simulink model "Watermark"  (R2021a)
settings: Solver=VariableStepAuto  StartTime=0.0  StopTime=tsim  RelTol=1e-3
values from neighbouring files (symbols this model uses):
  attack_DoS = 1    [main.m]
  attack_sat = 0    [main.m]
  delay = 700    [main.m]
  gamma1 = 0.70    (= 0.7)    [main.m]
  gamma2 = 0.60    (= 0.6)    [main.m]
  r1 = kc*h01    [main.m]
  r2 = kc*h02    [main.m]
  seuil_H0 = chi2inv(1-PFA, n_chi2 * timeWindow)    [main.m]
  SigmaInv = inv(Sigma)    [main.m]
  ta = 0.6*tsim    (= 1200)    [main.m]
undefined symbols (not defined in the file or in its folder): A1, a1, A2, a2, A3, a3, A4, a4, Adlin, Bdlin, C, Cdlin, g, K, k1, k2, L, m, n, sat_hmax, sat_hmin, sat_vmax, sat_vmin, sigma2_b, Ts, v01, v02, xd0
libraries: simulink x3, dspsrcs4 x2, commfilt2 x1
settings Model: Creator=aperodou  LastModifiedBy=Arthur
settings SolverCC: AlgebraicLoopSolver=TrustRegion
settings DebuggingCC: SFMachineParentedDataDiag=warning

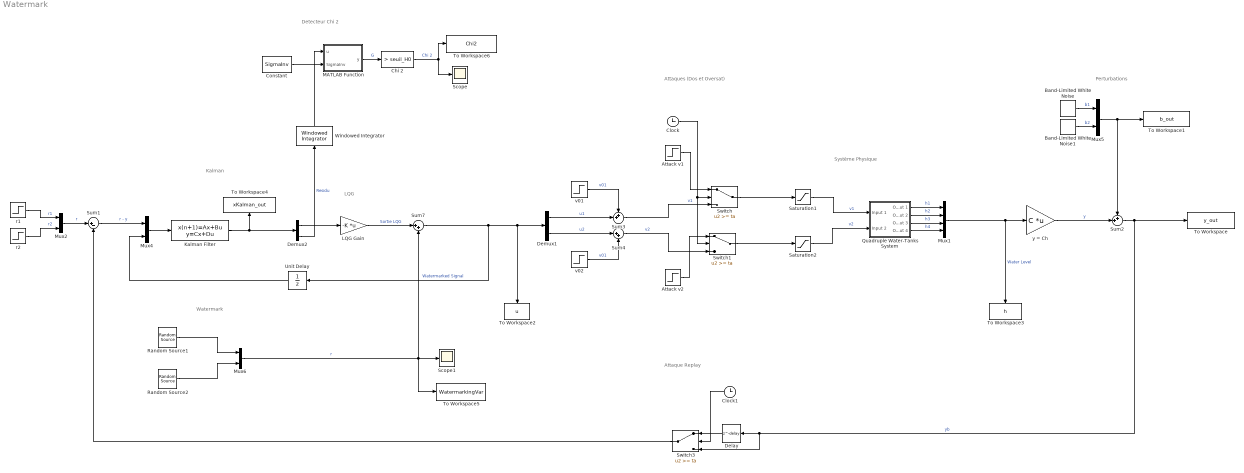
== system Watermark ==
  note: Attaques
      | (Dos et Oversat)
  note: Kalman
  note: Perturbations
  note: Système Physique
  note: Detecteur Chi 2
  note: LQG
  note: Attaque Replay
  note: Watermark
  Attack v1 : Step  Time=0  After=attack_DoS*0 + attack_sat*sat_vmax  SampleTime=0
  Attack v2 : Step  Time=0  After=attack_DoS*0 + attack_sat*sat_vmax  SampleTime=0
  Band-Limited White Noise : simulink/Sources/Band-Limited White Noise  Cov=[ sigma2_b ]  Ts=Ts  seed=[23341]
  Band-Limited White Noise1 : simulink/Sources/Band-Limited White Noise  Cov=[ sigma2_b]  Ts=Ts  seed=[20000]
  Chi 2 : simulink/Logic and Bit Operations/Compare To Constant  relop=>  const=seuil_H0  OutDataTypeStr=boolean
  Clock : Clock
  Clock1 : Clock
  Constant : Constant  Value=SigmaInv
  Delay : Delay  DelayLength=delay  InitialCondition=0
  Demux1 : Demux  Outputs=2
  Demux2 : Demux  Outputs=2
  Kalman Filter : DiscreteStateSpace  A=Adlin  B=[zeros(n,m) -Bdlin]  C=[eye(n) - L*Cdlin ; -Cdlin]  D=[L zeros(n,m) ; eye(m) zeros(m,m)]  InitialCondition=xd0  SampleTime=Ts
  LQG Gain : Gain  Gain=-K  Multiplication=Matrix(K*u) (u vector)
  MATLAB Function : MATLAB Function  TreatAsAtomicUnit=on
  Mux1 : Mux
  Mux{2,4..6} (4 alike) : Mux  Inputs=2
  Quadruple Water-Tanks System : Subsystem
  Random Source1 : dspsrcs4/Random Source  SrcType=Gaussian  NormMethod=Ziggurat  CltLength=12  MinVal=0  MaxVal=1  MeanVal=0  VarVal=varW  RepMode=Not repeatable  rawSeed=1  IsInherit=off  SampMode=Discrete  SampTime=1  SampFrame=1  DataType=Double  OutComplex=Real  OutputFrames=off
  Random Source2 : dspsrcs4/Random Source  SrcType=Gaussian  NormMethod=Ziggurat  CltLength=12  MinVal=0  MaxVal=1  MeanVal=0  VarVal=varW  RepMode=Not repeatable  rawSeed=1  IsInherit=off  SampMode=Discrete  SampTime=1  SampFrame=1  DataType=Double  OutComplex=Real  OutputFrames=off
  Saturation1 : Saturate  UpperLimit=sat_vmax  LowerLimit=sat_vmin
  Saturation2 : Saturate  UpperLimit=sat_vmax  LowerLimit=sat_vmin
  Scope : Scope
  Scope1 : Scope
  Sum1 : Sum  Inputs=|+-  SaturateOnIntegerOverflow=on
  Sum2 : Sum  Inputs=++|  SaturateOnIntegerOverflow=on
  Sum3 : Sum  Inputs=++|  SaturateOnIntegerOverflow=on
  Sum4 : Sum  Inputs=|++  SaturateOnIntegerOverflow=on
  Sum7 : Sum  Inputs=|++  SaturateOnIntegerOverflow=on
  Switch : Switch  Threshold=ta
  Switch1 : Switch  Threshold=ta
  Switch3 : Switch  Threshold=ta
  To Workspace : ToWorkspace  VariableName=y_out  SaveFormat=Timeseries  SampleTime=-1
  To Workspace1 : ToWorkspace  VariableName=b_out  SaveFormat=Timeseries  SampleTime=-1
  To Workspace2 : ToWorkspace  VariableName=u  SampleTime=-1
  To Workspace3 : ToWorkspace  VariableName=h  SampleTime=-1
  To Workspace4 : ToWorkspace  VariableName=xKalman_out  SaveFormat=Timeseries  SampleTime=-1
  To Workspace5 : ToWorkspace  VariableName=WatermarkingVar  SaveFormat=Timeseries  SampleTime=-1
  To Workspace6 : ToWorkspace  VariableName=Chi2  SampleTime=-1
  Unit Delay : UnitDelay  SampleTime=Ts  HasFrameUpgradeWarning=on
  Windowed Integrator : commfilt2/Windowed Integrator  integperiod=timeWindow  roundingMode=Floor  overflowMode=off  coeffDataTypeStr=Inherit: Same word length as input  coeffMin=[]  coeffMax=[]  coeffLastDataTypeStr=Inherit: Same word length as input  accumDataTypeStr=Inherit: Same as product output  accumLastDataTypeStr=Inherit: Same as product output  outputDataTypeStr=Inherit: Same as accumulator  outputMin=[]  outputMax=[]  outputLastDataTypeStr=Inherit: Same as accumulator
      settings: SourceProductBaseCode=CM
  r1 : Step  Time=0  After=r1  SampleTime=0
  r2 : Step  Time=0  After=r2  SampleTime=0
  v01 : Step  Time=0  After=v01  SampleTime=Ts
  v02 : Step  Time=0  After=v02  SampleTime=Ts
  y = Ch : Gain  Gain=C  Multiplication=Matrix(K*u) (u vector)
  wires:
  Quadruple Water-Tanks System/1(Output 1) -> Mux1/1  "h1"
  Quadruple Water-Tanks System/2(Output 2) -> Mux1/2  "h2"
  Quadruple Water-Tanks System/3(Output 3) -> Mux1/3  "h3"
  Quadruple Water-Tanks System/4(Output 4) -> Mux1/4  "h4"
  Mux1/1 -> y = Ch/1, To Workspace3/1  "Water Level"
  Mux2/1 -> Sum1/1  "r"
  Clock/1 -> Switch1/2, Switch/2
  Sum2/1 -> To Workspace/1, Switch3/3, Delay/1  "yb"
  y = Ch/1 -> Sum2/2  "y"
  r2/1 -> Mux2/2  "r2"
  r1/1 -> Mux2/1  "r1"
  Kalman Filter/1 -> Demux2/1, To Workspace4/1
  LQG Gain/1 -> Sum7/1  "Sortie LQG"
  Mux4/1 -> Kalman Filter/1
  Sum1/1 -> Mux4/1  "r - y"
  Unit Delay/1 -> Mux4/2
  Saturation1/1 -> Quadruple Water-Tanks System/1(Input 1)  "v1"
  Saturation2/1 -> Quadruple Water-Tanks System/2(Input 2)  "v2"
  v01/1 -> Sum3/1  "v01"
  Demux1/1 -> Sum3/2  "u1"
  Sum3/1 -> Switch/3  "v1"
  v02/1 -> Sum4/2  "v01"
  Demux1/2 -> Sum4/1  "u2"
  Sum4/1 -> Switch1/3  "v2"
  Band-Limited White Noise/1 -> Mux5/1  "b1"
  Band-Limited White Noise1/1 -> Mux5/2  "b2"
  Mux5/1 -> Sum2/1, To Workspace1/1
  Demux2/1 -> LQG Gain/1
  Constant/1 -> MATLAB Function/2(SigmaInv)
  MATLAB Function/1(y) -> Chi 2/1  "G"
  Demux2/2 -> Windowed Integrator/1  "Residu"
  Chi 2/1 -> To Workspace6/1, Scope/1  "Chi 2"
  Delay/1 -> Switch3/1
  Clock1/1 -> Switch3/2
  Attack v1/1 -> Switch/1
  Attack v2/1 -> Switch1/1
  Switch/1 -> Saturation1/1
  Switch1/1 -> Saturation2/1
  Switch3/1 -> Sum1/2
  Random Source1/1 -> Mux6/1
  Mux6/1 -> To Workspace5/1, Sum7/2, Scope1/1  "r"
  Random Source2/1 -> Mux6/2
  Sum7/1 -> Demux1/1, To Workspace2/1, Unit Delay/1  "Watermarked Signal"
  Windowed Integrator/1 -> MATLAB Function/1(u)

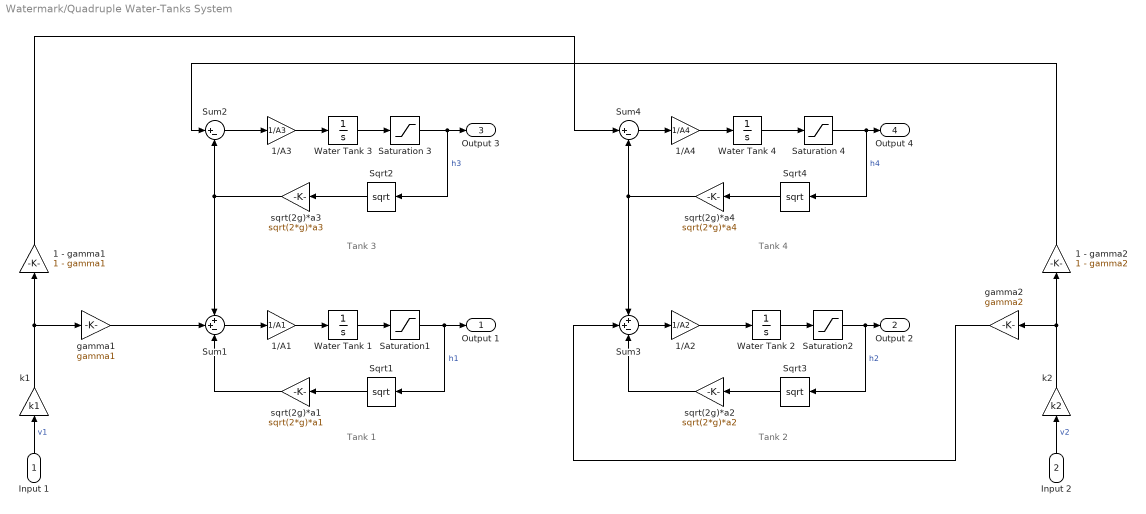
== system Watermark/Quadruple Water-Tanks System ==
  note: Tank 1
  note: Tank 3
  note: Tank 4
  note: Tank 2
  Input 1 : Inport
  Input 2 : Inport  Port=2
  1 - gamma1 : Gain  Gain=1 - gamma1  SaturateOnIntegerOverflow=on  OutDataTypeStr=Inherit: Same as input  ParamDataTypeStr=Inherit: Same as input
  1 - gamma2 : Gain  Gain=1 - gamma2  SaturateOnIntegerOverflow=on  OutDataTypeStr=Inherit: Same as input  ParamDataTypeStr=Inherit: Same as input
  1/A1 : Gain  Gain=1/A1  SaturateOnIntegerOverflow=on  OutDataTypeStr=Inherit: Same as input  ParamDataTypeStr=Inherit: Same as input
  1/A2 : Gain  Gain=1/A2  SaturateOnIntegerOverflow=on  OutDataTypeStr=Inherit: Same as input  ParamDataTypeStr=Inherit: Same as input
  1/A3 : Gain  Gain=1/A3  SaturateOnIntegerOverflow=on  OutDataTypeStr=Inherit: Same as input  ParamDataTypeStr=Inherit: Same as input
  1/A4 : Gain  Gain=1/A4  SaturateOnIntegerOverflow=on  OutDataTypeStr=Inherit: Same as input  ParamDataTypeStr=Inherit: Same as input
  Saturation 3 : Saturate  UpperLimit=sat_hmax  LowerLimit=sat_hmin
  Saturation 4 : Saturate  UpperLimit=sat_hmax  LowerLimit=sat_hmin
  Saturation1 : Saturate  UpperLimit=sat_hmax  LowerLimit=sat_hmin
  Saturation2 : Saturate  UpperLimit=sat_hmax  LowerLimit=sat_hmin
  Sqrt{1..4} (4 alike) : Sqrt  SaturateOnIntegerOverflow=on
  Sum1 : Sum  Inputs=++-  SaturateOnIntegerOverflow=on
  Sum2 : Sum  Inputs=|+-  SaturateOnIntegerOverflow=on
  Sum3 : Sum  Inputs=++-  SaturateOnIntegerOverflow=on
  Sum4 : Sum  Inputs=|+-  SaturateOnIntegerOverflow=on
  Water Tank {1..4} (4 alike) : Integrator
  gamma1 : Gain  Gain=gamma1  SaturateOnIntegerOverflow=on  OutDataTypeStr=Inherit: Same as input  ParamDataTypeStr=Inherit: Same as input
  gamma2 : Gain  Gain=gamma2  SaturateOnIntegerOverflow=on  OutDataTypeStr=Inherit: Same as input  ParamDataTypeStr=Inherit: Same as input
  k1 : Gain  Gain=k1  SaturateOnIntegerOverflow=on  OutDataTypeStr=Inherit: Same as input  ParamDataTypeStr=Inherit: Same as input
  k2 : Gain  Gain=k2  SaturateOnIntegerOverflow=on  OutDataTypeStr=Inherit: Same as input  ParamDataTypeStr=Inherit: Same as input
  sqrt(2g)*a1 : Gain  Gain=sqrt(2*g)*a1  SaturateOnIntegerOverflow=on  OutDataTypeStr=Inherit: Same as input  ParamDataTypeStr=Inherit: Same as input
  sqrt(2g)*a2 : Gain  Gain=sqrt(2*g)*a2  SaturateOnIntegerOverflow=on  OutDataTypeStr=Inherit: Same as input  ParamDataTypeStr=Inherit: Same as input
  sqrt(2g)*a3 : Gain  Gain=sqrt(2*g)*a3  SaturateOnIntegerOverflow=on  OutDataTypeStr=Inherit: Same as input  ParamDataTypeStr=Inherit: Same as input
  sqrt(2g)*a4 : Gain  Gain=sqrt(2*g)*a4  SaturateOnIntegerOverflow=on  OutDataTypeStr=Inherit: Same as input  ParamDataTypeStr=Inherit: Same as input
  Output 1 : Outport  VectorParamsAs1DForOutWhenUnconnected=off
  Output 2 : Outport  Port=2  VectorParamsAs1DForOutWhenUnconnected=off
  Output 3 : Outport  Port=3  VectorParamsAs1DForOutWhenUnconnected=off
  Output 4 : Outport  Port=4  VectorParamsAs1DForOutWhenUnconnected=off
  wires:
  Saturation2/1 -> Sqrt3/1, Output 2/1  "h2"
  Water Tank 2/1 -> Saturation2/1
  Water Tank 4/1 -> Saturation 4/1
  1/A1/1 -> Water Tank 1/1
  Sqrt2/1 -> sqrt(2g)*a3/1
  Saturation1/1 -> Sqrt1/1, Output 1/1  "h1"
  Water Tank 3/1 -> Saturation 3/1
  sqrt(2g)*a3/1 -> Sum2/2, Sum1/1
  sqrt(2g)*a4/1 -> Sum4/2, Sum3/1
  Saturation 3/1 -> Sqrt2/1, Output 3/1  "h3"
  Saturation 4/1 -> Sqrt4/1, Output 4/1  "h4"
  1/A4/1 -> Water Tank 4/1
  Water Tank 1/1 -> Saturation1/1
  Sum1/1 -> 1/A1/1
  Sqrt3/1 -> sqrt(2g)*a2/1
  k1/1 -> 1 - gamma1/1, gamma1/1
  Sqrt4/1 -> sqrt(2g)*a4/1
  k2/1 -> 1 - gamma2/1, gamma2/1
  Sum4/1 -> 1/A4/1
  gamma1/1 -> Sum1/2
  1 - gamma1/1 -> Sum4/1
  Input 2/1 -> k2/1  "v2"
  sqrt(2g)*a2/1 -> Sum3/3
  sqrt(2g)*a1/1 -> Sum1/3
  Sum2/1 -> 1/A3/1
  gamma2/1 -> Sum3/2
  1 - gamma2/1 -> Sum2/1
  1/A2/1 -> Water Tank 2/1
  Sum3/1 -> 1/A2/1
  1/A3/1 -> Water Tank 3/1
  Sqrt1/1 -> sqrt(2g)*a1/1
  Input 1/1 -> k1/1  "v1"

== matlab function Watermark/MATLAB Function ==
  data: u input; y output; SigmaInv input
function y = fcn(u,SigmaInv)

y = u'*SigmaInv*u;

end
